simulink model "gm_testing_interface"  (R2017a)
settings: Solver=FixedStepAuto  StartTime=0.0  StopTime=inf  RelTol=1e-3  EnableMultiTasking=on
undefined symbols (not defined in the file or in its folder): AXI4, Lite
libraries: axiinterfacelib x4, simulink x1
settings Model: SimulationMode=external  Creator=hyang344  LastModifiedBy=hyang344
settings SolverCC: EnableConcurrentExecution=on  ConcurrentTasks=on  PositivePriorityOrder=on  AutoInsertRateTranBlk=on
settings OptimizationCC: BlockReduction=off  ConditionallyExecuteInputs=off  PassReuseOutputArgsAs=Individual arguments  MaxStackSize=64
settings DebuggingCC: AlgebraicLoopMsg=error  SingleTaskRateTransMsg=error  ParameterTunabilityLossMsg=error
settings HardwareCC: ProdBitPerPointer=32  ProdBitPerSizeT=32  ProdBitPerPtrDiffT=32  ProdLargestAtomicInteger=Long  ProdLargestAtomicFloat=Double  ProdWordSize=32  ProdHWDeviceType=ARM Compatible->ARM Cortex  TargetEndianess=LittleEndian
settings SFSimCC: MATLABDynamicMemAlloc=off
settings RTWCC: SystemTargetFile=ert.tlc  HardwareBoard=ZedBoard  TLCOptions="-aInlineSetEventsForThisBaseRateFcn=TLC_FALSE -aSuppressMultiTaskScheduler=TLC_FALSE  -aRateBasedStepFcn=0"  TemplateMakefile=ert_default_tmf  Description=Embedded Coder  GenerateReport=on  Toolchain=Xilinx Software Development Kit (SDK)  IncludeHyperlinkInReport=on  LaunchReport=on  GenerateTraceInfo=on  GenerateTraceReport=on  GenerateTraceReportSl=on  GenerateTraceReportSf=on  GenerateTraceReportEml=on
settings CodeAppCC: ForceParamTrailComments=on  IgnoreCustomStorageClasses=off  OperatorAnnotations=on  SimulinkDataObjDesc=on  SFDataObjDesc=on  MATLABFcnDesc=on  InsertBlockDesc=on  MATLABSourceComments=on

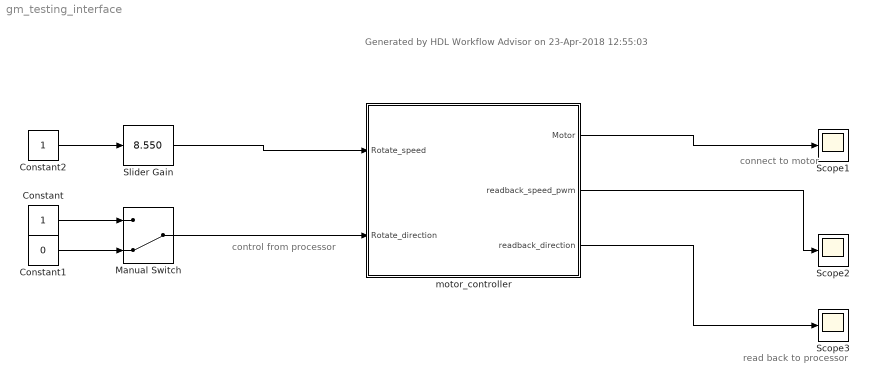
== system gm_testing_interface ==
  note: read back to
      | processor
  note: connect to
      | motor
  note: control from
      | processor
  note: Generated by HDL Workflow Advisor on 23-Apr-2018 12:55:03
  Constant : Constant  OutDataTypeStr=boolean
  Constant1 : Constant  Value=0  OutDataTypeStr=boolean
  Constant2 : Constant  OutDataTypeStr=fixdt(0, 4, 0)  SampleTime=0.01
  Manual Switch : ManualSwitch  CurrentSetting=0
  Scope1 : Scope
  Scope2 : Scope
  Scope3 : Scope
  Slider Gain : simulink/Math Operations/Slider Gain  gain=8.550  low=0  high=15
  motor_controller : Subsystem  TreatAsAtomicUnit=on  mask(AXI4-Lite/AXI4 Interface){}
      mask help:
      | This is an automatically generated subsystem block.
      | This contains the AXI interface blocks that communicate with the motor_con_ip IPCore generated from testing/motor_controller subsystem.
      mask Display: disp(sprintf('Xilinx Zynq \nAXI Interface'));
  wires:
  motor_controller/3("readback_direction ") -> Scope3/1
  motor_controller/2(readback_speed_pwm) -> Scope2/1
  Manual Switch/1 -> motor_controller/2(Rotate_direction)
  Constant/1 -> Manual Switch/1
  motor_controller/1(Motor) -> Scope1/1
  Constant2/1 -> Slider Gain/1
  Slider Gain/1 -> motor_controller/1(Rotate_speed)
  Constant1/1 -> Manual Switch/2

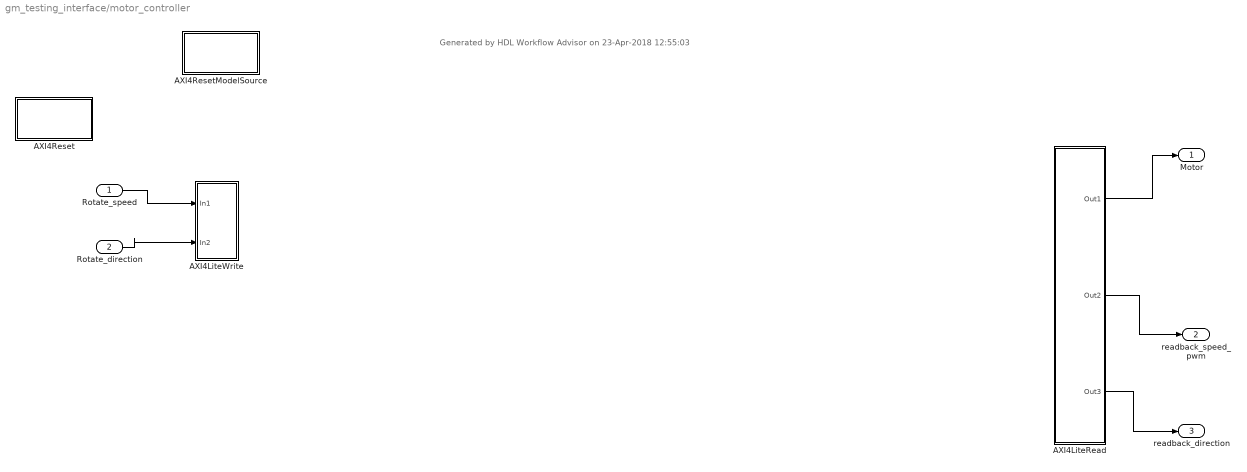
== system gm_testing_interface/motor_controller ==
  note: Generated by HDL Workflow Advisor on 23-Apr-2018 12:55:03
  Rotate_speed : Inport  OutDataTypeStr=fixdt(0, 4, 0)
  Rotate_direction : Inport  Port=2  OutDataTypeStr=boolean
  AXI4LiteRead : Subsystem  Priority=10
  AXI4LiteWrite : Subsystem  Priority=1
  AXI4Reset : Subsystem  mask(System Start){ShowInLibBrowser=0}
      mask prompts: ShowInLibBrowser "Simulink:masks:CustCodeMaskParam1_MP"
      settings: CopyFcn=cccopyfcn(gcb)  OpenFcn=ccopenfcn('System Start Function')
      mask Help: eval('feval(''rtwprivate'',''rtwhelpview'',''rtw_sys_start_block'')');
      mask Display: disp('System\nStart');
  AXI4ResetModelSource : Subsystem  mask(Model Source){ShowInLibBrowser=0}
      mask prompts: ShowInLibBrowser "Simulink:masks:CustCodeMaskParam1_MP"
      settings: CopyFcn=cccopyfcn(gcb)  OpenFcn=ccopenfcn('Model Source')
      mask Help: eval('feval(''rtwprivate'',''rtwhelpview'',''rtw_model_source_block'')');
      mask Display: disp('Model\nSource');
  Motor : Outport
  readback_speed_pwm : Outport  Port=2
  "readback_direction " : Outport  Port=3
  wires:
  Rotate_speed/1 -> AXI4LiteWrite/1(In1)
  Rotate_direction/1 -> AXI4LiteWrite/2(In2)
  AXI4LiteRead/1(Out1) -> Motor/1
  AXI4LiteRead/2(Out2) -> readback_speed_pwm/1
  AXI4LiteRead/3(Out3) -> "readback_direction "/1

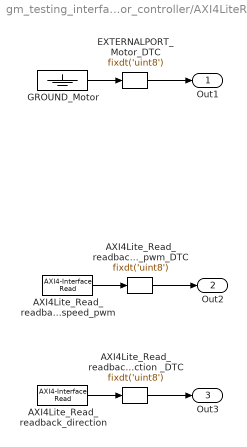
== system gm_testing_interface/motor_controller/AXI4LiteRead ==
  "AXI4Lite_Read_readback_direction " : axiinterfacelib/AXI4-Interface Read  Priority=4  AXIInterfaceType=AXI4-Lite  DeviceName=/dev/mwipcore  RegisterOffset=hex2dec('10C')  DataLength=1  DataType=uint32  SampleTime=-1  blockPlatform=ZYNQ  SimulateUsing=Interpreted Execution
      settings: SourceProductName=Embedded Coder Support Package for Xilinx Zynq-7000 Platform  SourceProductBaseCode=ECZYNQ7000
  AXI4Lite_Read_readback_direction _DTC : DataTypeConversion  OutDataTypeStr=fixdt('uint8')  ConvertRealWorld=Stored Integer (SI)
  AXI4Lite_Read_readback_speed_pwm : axiinterfacelib/AXI4-Interface Read  Priority=3  AXIInterfaceType=AXI4-Lite  DeviceName=/dev/mwipcore  RegisterOffset=hex2dec('108')  DataLength=1  DataType=uint32  SampleTime=-1  blockPlatform=ZYNQ  SimulateUsing=Interpreted Execution
      settings: SourceProductName=Embedded Coder Support Package for Xilinx Zynq-7000 Platform  SourceProductBaseCode=ECZYNQ7000
  AXI4Lite_Read_readback_speed_pwm_DTC : DataTypeConversion  OutDataTypeStr=fixdt('uint8')  ConvertRealWorld=Stored Integer (SI)
  EXTERNALPORT_Motor_DTC : DataTypeConversion  OutDataTypeStr=fixdt('uint8')
  GROUND_Motor : Ground
  Out1 : Outport
  Out2 : Outport  Port=2
  Out3 : Outport  Port=3
  wires:
  "AXI4Lite_Read_readback_direction "/1 -> AXI4Lite_Read_readback_direction _DTC/1
  AXI4Lite_Read_readback_direction _DTC/1 -> Out3/1
  AXI4Lite_Read_readback_speed_pwm_DTC/1 -> Out2/1
  AXI4Lite_Read_readback_speed_pwm/1 -> AXI4Lite_Read_readback_speed_pwm_DTC/1
  GROUND_Motor/1 -> EXTERNALPORT_Motor_DTC/1
  EXTERNALPORT_Motor_DTC/1 -> Out1/1

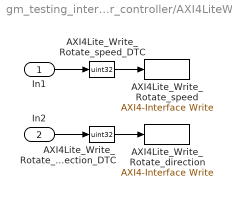
== system gm_testing_interface/motor_controller/AXI4LiteWrite ==
  In1 : Inport
  In2 : Inport  Port=2
  AXI4Lite_Write_Rotate_direction : axiinterfacelib/AXI4-Interface Write  Priority=2  AXIInterfaceType=AXI4-Lite  DeviceName=/dev/mwipcore  RegisterOffset=hex2dec('104')  blockPlatform=ZYNQ  SimulateUsing=Interpreted execution
      settings: SourceProductName=Embedded Coder Support Package for Xilinx Zynq-7000 Platform  SourceProductBaseCode=ECZYNQ7000
  AXI4Lite_Write_Rotate_direction_DTC : DataTypeConversion  OutDataTypeStr=uint32  ConvertRealWorld=Stored Integer (SI)
  AXI4Lite_Write_Rotate_speed : axiinterfacelib/AXI4-Interface Write  Priority=1  AXIInterfaceType=AXI4-Lite  DeviceName=/dev/mwipcore  RegisterOffset=hex2dec('100')  blockPlatform=ZYNQ  SimulateUsing=Interpreted execution
      settings: SourceProductName=Embedded Coder Support Package for Xilinx Zynq-7000 Platform  SourceProductBaseCode=ECZYNQ7000
  AXI4Lite_Write_Rotate_speed_DTC : DataTypeConversion  OutDataTypeStr=uint32  ConvertRealWorld=Stored Integer (SI)
  wires:
  In1/1 -> AXI4Lite_Write_Rotate_speed_DTC/1
  AXI4Lite_Write_Rotate_speed_DTC/1 -> AXI4Lite_Write_Rotate_speed/1
  In2/1 -> AXI4Lite_Write_Rotate_direction_DTC/1
  AXI4Lite_Write_Rotate_direction_DTC/1 -> AXI4Lite_Write_Rotate_direction/1

== system gm_testing_interface/motor_controller/AXI4Reset ==

== system gm_testing_interface/motor_controller/AXI4ResetModelSource ==
